simulink model "equation_5"  (R2018b)
settings: Solver=VariableStepAuto  StartTime=0.0  StopTime=100  RelTol=1e-3
settings Model: Creator=dinet  LastModifiedBy=dinet

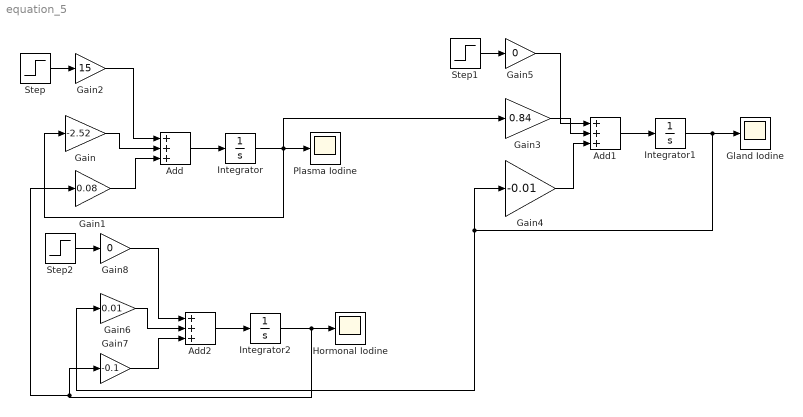
== system equation_5 ==
  Add : Sum  Inputs=+++
  Add1 : Sum  Inputs=+++
  Add2 : Sum  Inputs=+++
  Gain : Gain  Gain=-2.52
  Gain1 : Gain  Gain=0.08
  Gain2 : Gain  Gain=15
  Gain3 : Gain  Gain=0.84
  Gain4 : Gain  Gain=-0.01
  Gain5 : Gain  Gain=0
  Gain6 : Gain  Gain=0.01
  Gain7 : Gain  Gain=-0.1
  Gain8 : Gain  Gain=0
  Gland Iodine : Scope
  Hormonal Iodine : Scope
  Integrator : Integrator  InitialCondition=81.2
  Integrator1 : Integrator  InitialCondition=6821
  Integrator2 : Integrator  InitialCondition=682.1
  Plasma Iodine : Scope
  Step : Step  Time=0  SampleTime=0
  Step1 : Step  Time=0  SampleTime=0
  Step2 : Step  Time=0  SampleTime=0
  wires:
  Step/1 -> Gain2/1
  Step1/1 -> Gain5/1
  Step2/1 -> Gain8/1
  Gain2/1 -> Add/1
  Integrator/1 -> Gain3/1, Gain/1, Plasma Iodine/1
  Add/1 -> Integrator/1
  Gain/1 -> Add/2
  Gain8/1 -> Add2/1
  Integrator2/1 -> Gain1/1, Gain7/1, Hormonal Iodine/1
  Add2/1 -> Integrator2/1
  Gain7/1 -> Add2/3
  Gain1/1 -> Add/3
  Integrator1/1 -> Gain6/1, Gain4/1, Gland Iodine/1
  Gain4/1 -> Add1/3
  Gain6/1 -> Add2/2
  Gain3/1 -> Add1/2
  Gain5/1 -> Add1/1
  Add1/1 -> Integrator1/1
